simulink model "PIDRelayy"  (R2021b)
settings: Solver=FixedStepAuto  StartTime=0.0  StopTime=1000  FixedStep=0.2  RelTol=1e-3
settings Model: Creator=ismt  LastModifiedBy=ismt

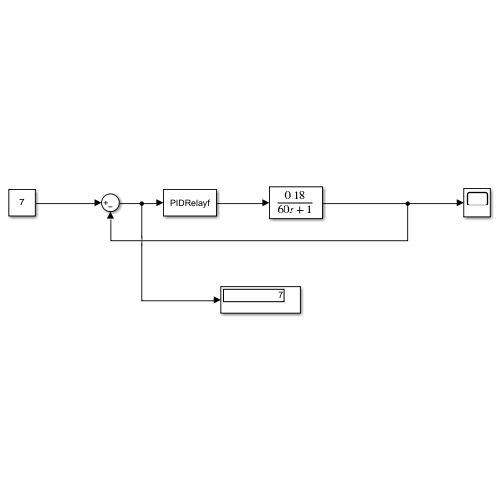
[thumbnail: Simulink's stored preview of the top-level diagram]
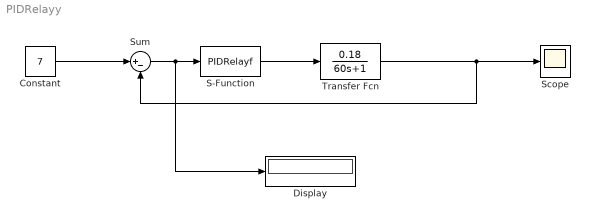
== system PIDRelayy ==
  Constant : Constant  Value=7
  Display : Display
  S-Function : S-Function  FunctionName=PIDRelayf  SFunctionDeploymentMode=off  EnableBusSupport=off
  Scope : Scope
  Sum : Sum  Inputs=|+-
  Transfer Fcn : TransferFcn  Numerator=[0.18]  Denominator=[60 1]
  wires:
  S-Function/1 -> Transfer Fcn/1
  Sum/1 -> Display/1, S-Function/1
  Constant/1 -> Sum/1
  Transfer Fcn/1 -> Sum/2, Scope/1
